simulink model "JenaFox_NCm"  (R2018a)
settings: Solver=ode23s  StartTime=0.0  StopTime=20  MaxStep=maxStep  RelTol=1e-3  AbsTol=absTol
values from neighbouring files (symbols this model uses):
  amplifier = 2.28    [init_motor_parameters.m]
  c_coupling_hip = 7/hip_Ra*hip_k/hip_i    (= 1.22844788155)    [init_motor_parameters.m]
  c_coupling_knee = 7/knee_Ra*knee_k/knee_i    (= 0.698088436179)    [init_motor_parameters.m]
  c_hs = 0.1    [Fox_param.m]
  d_coupling_knee = 0.5    [init_motor_parameters.m]
  d_hs = 0.35    [Fox_param.m]
  g = 9.80665    [Fox_param.m]    (also in init_motor_parameters.m = 9.81)
  hip_i = 1/300.4858    (= 0.00332794428223)    [init_motor_parameters.m]
  hip_Jm = 1/2*hip_m*hip_r^2    (= 1e-07)    [init_motor_parameters.m]
  hip_k = (hip_Um-hip_I0*hip_Ra)*60/(2*pi*hip_n0)    (= 0.00320895298542)    [init_motor_parameters.m]
  hip_Mrg = hip_k*hip_I0g    (= 0.000320895298542)    [init_motor_parameters.m]
  hip_Mrhg = hip_k*hip_Iag    (= 0.000381865405265)    [init_motor_parameters.m]
  hip_na = (hip_Us-(hip_I0*hip_Ra))/hip_k    (= 105.13168591)    [init_motor_parameters.m]
  hip_Ra = hip_Um/hip_Is    (= 5.49450549451)    [init_motor_parameters.m]
  IC_motor_hip_l = deg2rad(IC_phi_hip_l/hip_i)    [init_motor_parameters.m]
  IC_motor_hip_r = deg2rad(IC_phi_hip_r/hip_i)    [init_motor_parameters.m]
  IC_motor_knee_l = deg2rad(IC_phi_knee_l/knee_i)    [init_motor_parameters.m]
  IC_motor_knee_r = deg2rad(IC_phi_knee_r/knee_i)    [init_motor_parameters.m]
  IC_phi_hip_l = 10    [Fox_param.m]
  IC_phi_hip_r = -29    [Fox_param.m]
  IC_v_motor_hip = 0    [init_motor_parameters.m]
  IC_v_motor_knee = 0    [init_motor_parameters.m]
  k_gx = 10*M_RB/0.01    [Fox_param.m]
  k_gy = 150*M_RB/0.01    [Fox_param.m]
  knee_i = 1/185.8428    (= 0.00538089180748)    [init_motor_parameters.m]
  knee_Jm = 1/2*knee_m*knee_r^2    (= 3.2e-08)    [init_motor_parameters.m]
  knee_k = (knee_Um-knee_I0*knee_Ra)*60/(2*pi*knee_n0)    (= 0.000596244182085)    [init_motor_parameters.m]
  knee_Mrg = knee_k*knee_I0g    (= 6.55868600293e-05)    [init_motor_parameters.m]
  knee_Mrhg = knee_k*knee_Iag    (= 9.59953133156e-05)    [init_motor_parameters.m]
  knee_na = (knee_Us-knee_I0*knee_Ra)/knee_k    (= 1360.36733855)    [init_motor_parameters.m]
  knee_Ra = knee_Um/knee_Is    (= 1.11111111111)    [init_motor_parameters.m]
  mu_slide = 4.6    [Fox_param.m]
  mu_stick = 0.8    [Fox_param.m]
  v_gx_max = 0.06    [Fox_param.m]
  v_gy_max = 0.70    (= 0.7)    [Fox_param.m]
  vLimit = 0.01    [Fox_param.m]
undefined symbols (not defined in the file or in its folder): param, smiData, X, Y, Z
libraries: sm_lib x38, nesl_utility x32, simulink x22, simulink_extras x8
(part 1 of 3)
settings Model: SimulationMode=accelerator  Creator=Work  LastModifiedBy=Work
settings RTWCC: Toolchain=MinGW64 | gmake (64-bit Windows)
settings ExplorerConfigSet: SimMechanicsOpenEditorOnUpdate=off  InternalSimMechanicsExplorerSettings="<ExplorerConfiguration><canonicalview>default</canonicalview><AnimationSetting><BasePlaybackSpeed>1.0</BasePlaybackSpeed><PlaybackSpeedFactor>0.0625</PlaybackSpeedFactor></AnimationSetting><TilePanel><TileInfo><Tiles Columns=\"1\" Count=\"1\" Rows=\"1\"><Column Weight=\"1\"/><Row Weight=\"1\"/><Tile Height=\"1\" Width=\"1\" X=\"0\" Y=\"0\"/></Tiles></TileInfo><SceneInfo><SceneViewer><BGColor><R>1</R><G>1</G><B>1</B></BGColor><Camera><DoPerspective>on</DoPerspective><Position><X>-4.33680868994201774e-19</X><Y>0.187999999999999973</Y><Z>0.5</Z></Position><Center><X>-4.33680868994201774e-19</X><Y>0.187999999999999973</Y><Z>-0.5</Z></Center><Up><X>0</X><Y>1</Y><Z>0</Z></Up><ViewLimDist>1</ViewLimDist><YLim>0.466307658154998583</YLim><XLim>0.581939865120500666</XLim></Camera></SceneViewer></SceneInfo></TilePanel><MechEditorPanel><Cameras><Camera><Id>Camera1</Id><Value><Name>Camera1</Name><NativeCamera><PositionTrackingFeature>Subsystem.Camera.Frame1</PositionTrackingFeature><CenterTrackingFeature>Subsystem.Camera.Frame1</CenterTrackingFeature><UpVectorTrackingFeature>Subsystem.Camera.Frame1</UpVectorTrackingFeature><CenterTrackingOrigin>off</CenterTrackingOrigin><CenterTrackingDirection>-Z</CenterTrackingDirection><UpVectorTrackingDirection>+Y</UpVectorTrackingDirection></NativeCamera></Value></Camera></Cameras><GfxPanelCameraMap><MapElement CameraMLId=\"Camera1\" GfxPanelIndex=\"0\"/></GfxPanelCameraMap><VideoCreator><PlaybackSpeedRatio>1.0</PlaybackSpeedRatio><FrameRate>30</FrameRate><VideoFormat>Motion JPEG AVI</VideoFormat><FrameSize>auto</FrameSize></VideoCreator></MechEditorPanel></ExplorerConfiguration>"

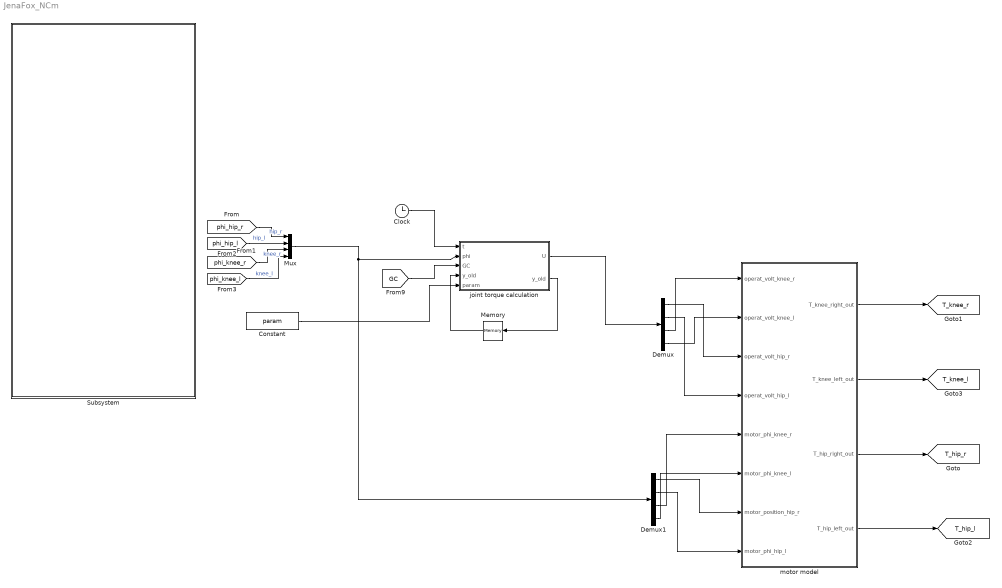
== system JenaFox_NCm ==
  Clock : Clock
  Constant : Constant  Value=param
  Demux : Demux
  Demux1 : Demux
  Memory : Memory  InitialCondition=[0 0;0 0;0 0;0 0;0 0]
  Mux : Mux
  Subsystem : Subsystem
      mask Display: image('robot_new.png');
  joint torque calculation : MATLAB Function  TreatAsAtomicUnit=on  SystemSampleTime=1e-3
  motor model : Subsystem
  tag scope: T_hip_l=global, T_hip_r=global, T_knee_l=global, T_knee_r=global
  wires:
  motor model/2(T_knee_left_out) -> [T_knee_l]
  motor model/1(T_knee_right_out) -> [T_knee_r]
  motor model/4(T_hip_left_out) -> [T_hip_l]
  motor model/3(T_hip_right_out) -> [T_hip_r]
  [phi_knee_l] -> Mux/4  "knee_l"
  [phi_hip_r] -> Mux/1  "hip_r"
  Mux/1 -> joint torque calculation/2(phi), Demux1/1
  [phi_hip_l] -> Mux/2  "hip_l"
  [phi_knee_r] -> Mux/3  "knee_r"
  Demux1/1 -> motor model/7(motor_position_hip_r)
  Demux1/2 -> motor model/8(motor_phi_hip_l)
  Demux1/3 -> motor model/5(motor_phi_knee_r)
  Demux1/4 -> motor model/6(motor_phi_knee_l)
  joint torque calculation/1(U) -> Demux/1
  Demux/1 -> motor model/3(operat_volt_hip_r)
  Demux/2 -> motor model/4(operat_volt_hip_l)
  Demux/3 -> motor model/1(operat_volt_knee_r)
  Demux/4 -> motor model/2(operat_volt_knee_l)
  Clock/1 -> joint torque calculation/1(t)
  [GC] -> joint torque calculation/3(GC)
  joint torque calculation/2(y_old) -> Memory/1
  Memory/1 -> joint torque calculation/4("y_old ")
  Constant/1 -> joint torque calculation/5(param)

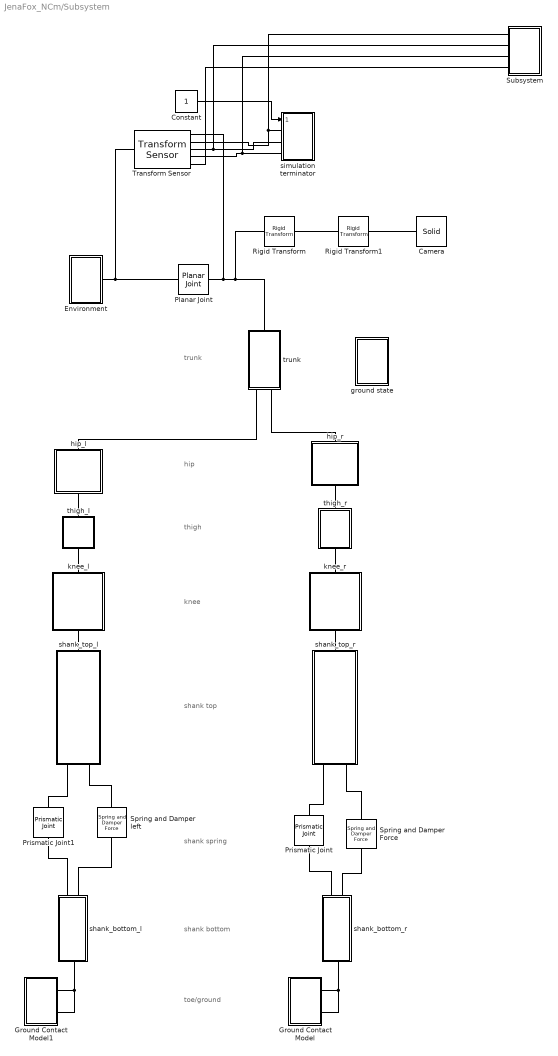
== system JenaFox_NCm/Subsystem ==
  note: trunk
  note: hip
  note: thigh
  note: knee
  note: shank top
  note: shank spring
  note: shank bottom
  note: toe/ground
  Camera : sm_lib/Body Elements/Solid  InertiaType=Custom  Mass=0  MassUnits=kg  CenterOfMass=[0 0 0]  CenterOfMassUnits=m  MomentsOfInertia=[0 0 0]  MomentsOfInertiaUnits=kg*m^2  ProductsOfInertia=[0 0 0]  ProductsOfInertiaUnits=kg*m^2  DensityBased=on  Density=1000  DensityUnits=kg/m^3  DoExposeReferenceFrame=off  SerializedFrames=<Frames><Frame><Id>Frame1</Id><Value><Name>F1</Name><Origin><Source>CenterOfMassFrame</Source><FeatureName></FeatureName></Origin><PrimaryAxis><DefinedDirection>+Z</DefinedDirection><Source>ReferenceFrame</Source><SourceDirection>+Z</SourceDirection><FeatureName></FeatureName></PrimaryAxis><SecondaryAxis><DefinedDirection>+X</DefinedDirection><Source>ReferenceFrame</Source><SourceDirection>+X</SourceDirection><FeatureName></FeatureName></SecondaryAxis></Value></Frame></Frames>  GraphicType=FromGeometry  MarkerShape=Sphere  MarkerSize=10  GraphicVisPropType=SimpleVisualProperties  GraphicDiffuseColor=[0.5 0.5 0.5]  GraphicSpecularColor=[0.5 0.5 0.5 1.0]  GraphicAmbientColor=[0.15 0.15 0.15 1.0]  GraphicEmissiveColor=[0.0 0.0 0.0 1.0]  GraphicShininess=75  GraphicOpacity=1.0  GeometryShape=Sphere  RectangleSize=[1 1]  RectangleSizeUnits=m  BrickDimensions=[1 1 1]  BrickDimensionUnits=m  CylinderRadius=1  CylinderRadiusUnits=m  CylinderLength=1  CylinderLengthUnits=m  SphereRadius=1e-6  SphereRadiusUnits=m  EllipsoidRadii=[1 1 1]  EllipsoidRadiiUnits=m  ExtrusionCrossSection=[1 1; -1 1; -1 -1; 1 -1]  ExtrusionCrossSectionUnits=m  ExtrusionLength=1  ExtrusionLengthUnits=m  PolygonNumSides=3  PolygonOuterRadius=1  PolygonOuterRadiusUnits=m  ExtGeomFileType=STEP  ExtGeomFileUnits=m  RevolutionCrossSection=[1 1; 1 -1; 2 -1; 2 1]  RevolutionCrossSectionUnits=m  RevolutionExtent=Full  RevolutionAngle=180  RevolutionAngleUnits=deg
  Constant : Constant
  Environment : Subsystem
  Ground Contact Model : Subsystem
  Ground Contact Model1 : Subsystem
  Planar Joint : sm_lib/Joints/Planar Joint  SenseConstraintForce=off  SenseConstraintForceX=off  SenseConstraintForceY=off  SenseConstraintForceZ=off  SenseConstraintTorque=off  SenseConstraintTorqueX=off  SenseConstraintTorqueY=off  SenseConstraintTorqueZ=off  SenseTotalForce=off  SenseTotalForceX=off  SenseTotalForceY=off  SenseTotalForceZ=off  SenseTotalTorque=off  SenseTotalTorqueX=off  SenseTotalTorqueY=off  SenseTotalTorqueZ=off  CompositeWrenchDir=FollowerOnBase  CompositeWrenchFrame=BaseFrame  PxEquilibriumPosition=0  PxEquilibriumPositionUnits=m  PxSpringStiffness=0  PxSpringStiffnessUnits=N/m  PxDampingCoefficient=0  PxDampingCoefficientUnits=N/(m/s)  PxTorqueActuationMode=NoTorque  PxMotionActuationMode=ComputedMotion  PxSensePosition=off  PxSenseVelocity=off  PxSenseAcceleration=off  PxSenseTorqueForce=off  PxPositionTargetSpecify=off  PxPositionTargetPriority=High  PxPositionTargetValue=0  PxPositionTargetValueUnits=m  PxVelocityTargetSpecify=on  PxVelocityTargetPriority=High  PxVelocityTargetValue=IC_vCOM_x  PxVelocityTargetValueUnits=m/s  PyEquilibriumPosition=0  PyEquilibriumPositionUnits=m  PySpringStiffness=0  PySpringStiffnessUnits=N/m  PyDampingCoefficient=0  PyDampingCoefficientUnits=N/(m/s)  PyTorqueActuationMode=NoTorque  PyMotionActuationMode=ComputedMotion  PySensePosition=off  PySenseVelocity=off  PySenseAcceleration=off  PySenseTorqueForce=off  PyPositionTargetSpecify=on  PyPositionTargetPriority=High  PyPositionTargetValue=IC_y  PyPositionTargetValueUnits=m  PyVelocityTargetSpecify=on  PyVelocityTargetPriority=High  PyVelocityTargetValue=IC_vCOM_y  PyVelocityTargetValueUnits=m/s  RzEquilibriumPosition=0  RzEquilibriumPositionUnits=deg  RzSpringStiffness=500  RzSpringStiffnessUnits=N*m/deg  RzDampingCoefficient=5  RzDampingCoefficientUnits=N*m/(deg/s)  RzTorqueActuationMode=NoTorque  RzMotionActuationMode=ComputedMotion  RzSensePosition=off  RzSenseVelocity=off  RzSenseAcceleration=off  RzSenseTorqueForce=off  RzPositionTargetSpecify=on  RzPositionTargetPriority=High  RzPositionTargetValue=0  RzPositionTargetValueUnits=deg  RzVelocityTargetSpecify=on  RzVelocityTargetPriority=High  RzVelocityTargetValue=0  RzVelocityTargetValueUnits=deg/s
  Prismatic Joint : sm_lib/Joints/Prismatic Joint  SenseConstraintForce=off  SenseConstraintForceX=off  SenseConstraintForceY=off  SenseConstraintForceZ=off  SenseConstraintTorque=off  SenseConstraintTorqueX=off  SenseConstraintTorqueY=off  SenseConstraintTorqueZ=off  SenseTotalForce=off  SenseTotalForceX=off  SenseTotalForceY=off  SenseTotalForceZ=off  SenseTotalTorque=off  SenseTotalTorqueX=off  SenseTotalTorqueY=off  SenseTotalTorqueZ=off  CompositeWrenchDir=FollowerOnBase  CompositeWrenchFrame=BaseFrame  EquilibriumPosition=0  EquilibriumPositionUnits=m  SpringStiffness=0  SpringStiffnessUnits=N/m  DampingCoefficient=0  DampingCoefficientUnits=N/(m/s)  TorqueActuationMode=NoTorque  MotionActuationMode=ComputedMotion  SensePosition=off  SenseVelocity=off  SenseAcceleration=off  SenseTorqueForce=off  PositionTargetSpecify=off  PositionTargetPriority=High  PositionTargetValue=0  PositionTargetValueUnits=m  VelocityTargetSpecify=off  VelocityTargetPriority=High  VelocityTargetValue=0  VelocityTargetValueUnits=m/s
  Prismatic Joint1 : sm_lib/Joints/Prismatic Joint  SenseConstraintForce=off  SenseConstraintForceX=off  SenseConstraintForceY=off  SenseConstraintForceZ=off  SenseConstraintTorque=off  SenseConstraintTorqueX=off  SenseConstraintTorqueY=off  SenseConstraintTorqueZ=off  SenseTotalForce=off  SenseTotalForceX=off  SenseTotalForceY=off  SenseTotalForceZ=off  SenseTotalTorque=off  SenseTotalTorqueX=off  SenseTotalTorqueY=off  SenseTotalTorqueZ=off  CompositeWrenchDir=FollowerOnBase  CompositeWrenchFrame=BaseFrame  EquilibriumPosition=0  EquilibriumPositionUnits=m  SpringStiffness=0  SpringStiffnessUnits=N/m  DampingCoefficient=0  DampingCoefficientUnits=N/(m/s)  TorqueActuationMode=NoTorque  MotionActuationMode=ComputedMotion  SensePosition=off  SenseVelocity=off  SenseAcceleration=off  SenseTorqueForce=off  PositionTargetSpecify=off  PositionTargetPriority=High  PositionTargetValue=0  PositionTargetValueUnits=m  VelocityTargetSpecify=off  VelocityTargetPriority=High  VelocityTargetValue=0  VelocityTargetValueUnits=m/s
  Rigid Transform : sm_lib/Frames and Transforms/Rigid Transform  TranslationMethod=StandardAxis  TranslationStandardOffset=.5  TranslationLengthUnit=m  TranslationStandardAxis=+Z  TranslationCartesianOffset=[0 0 0]  TranslationROffset=0  TranslationROffsetUnits=m  TranslationZOffset=0  TranslationZOffsetUnits=m  TranslationThetaOffset=0  TranslationThetaOffsetUnits=deg  RotationMethod=None  RotationAngleUnits=deg  RotationStandardAxis=+Z  RotationAngle=0.0  RotationArbitraryAxis=[0 0 1]  FollAlignAxisA=+X  BaseAlignAxisA=+Y  FollAlignAxisB=+Y  BaseAlignAxisB=+Z  RotationSequenceAxes=FollowerAxes  RotationSequence=XYX  RotationSequenceAngles=[0 0 0]  RotationSequenceAnglesUnits=deg  RotationMatrix=[1 0 0; 0 1 0; 0 0 1]
  Rigid Transform1 : sm_lib/Frames and Transforms/Rigid Transform  TranslationMethod=StandardAxis  TranslationStandardOffset=.1  TranslationLengthUnit=m  TranslationStandardAxis=-Y  TranslationCartesianOffset=[0 0 0]  TranslationROffset=0  TranslationROffsetUnits=m  TranslationZOffset=0  TranslationZOffsetUnits=m  TranslationThetaOffset=0  TranslationThetaOffsetUnits=deg  RotationMethod=None  RotationAngleUnits=deg  RotationStandardAxis=+Z  RotationAngle=0.0  RotationArbitraryAxis=[0 0 1]  FollAlignAxisA=+X  BaseAlignAxisA=+Y  FollAlignAxisB=+Y  BaseAlignAxisB=+Z  RotationSequenceAxes=FollowerAxes  RotationSequence=XYX  RotationSequenceAngles=[0 0 0]  RotationSequenceAnglesUnits=deg  RotationMatrix=[1 0 0; 0 1 0; 0 0 1]
  Spring and Damper Force : sm_lib/Forces and Torques/Spring and Damper Force  NaturalLength=spring_ankle_rl_r  NaturalLengthUnits=m  SpringStiffness=spring_ankle_c_r  SpringStiffnessUnits=N/m  DampingCoefficient=damper_ankle_r  DampingCoefficientUnits=N/(m/s)  SenseForce=off
      settings: SourceProductName=Simscape Multibody
  Spring and Damper left : sm_lib/Forces and Torques/Spring and Damper Force  NaturalLength=spring_ankle_rl_l  NaturalLengthUnits=m  SpringStiffness=spring_ankle_c_l  SpringStiffnessUnits=N/m  DampingCoefficient=damper_ankle_l  DampingCoefficientUnits=N/(m/s)  SenseForce=off
      settings: SourceProductName=Simscape Multibody
  Subsystem : Subsystem
  Transform Sensor : sm_lib/Frames and Transforms/Transform Sensor  MeasurementFrame=World  SenseAngle=off  SenseAxis=off  SenseAngle1=off  SenseAngle2=off  SenseAngle3=off  SenseQ=off  SenseR=off  SenseOmegaX=off  SenseOmegaY=off  SenseOmegaZ=off  SenseOmega1=off  SenseOmega2=off  SenseOmega3=off  SenseQDot=off  SenseRDot=off  SenseAlphaX=off  SenseAlphaY=off  SenseAlphaZ=off  SenseAlpha1=off  SenseAlpha2=off  SenseAlpha3=off  SenseQDDot=off  SenseRDDot=off  SenseX=on  SenseY=on  SenseZ=off  SenseRad=off  SenseAzim=off  SenseDist=off  SenseInc=off  SenseXDot=on  SenseYDot=on  SenseZDot=off  SenseRadDot=off  SenseAzimDot=off  SenseDistDot=off  SenseIncDot=off  SenseXDDot=off  SenseYDDot=off  SenseZDDot=off  SenseRadDDot=off  SenseAzimDDot=off  SenseDistDDot=off  SenseIncDDot=off
  ground state : Subsystem
  hip_l : Subsystem
  hip_r : Subsystem
  knee_l : Subsystem
  knee_r : Subsystem
  shank_bottom_l : Subsystem
  shank_bottom_r : Subsystem
  shank_top_l : Subsystem
  shank_top_r : Subsystem
  simulation terminator : Subsystem
  thigh_l : Subsystem
  thigh_r : Subsystem
  trunk : Subsystem
  wires:
  Constant/1 -> simulation terminator/1(enable)
  connections:
  Spring and Damper Force/LConn1 -- shank_bottom_r/LConn2
  knee_r/RConn1 -- shank_top_r/LConn1
  hip_r/RConn1 -- thigh_r/LConn1
  knee_r/LConn1 -- thigh_r/RConn1
  Prismatic Joint1/LConn1 -- shank_bottom_l/LConn1
  hip_l/RConn1 -- thigh_l/LConn1
  Ground Contact Model/RConn1 -- Ground Contact Model/RConn2 -- shank_bottom_r/RConn1
  Prismatic Joint/RConn1 -- shank_top_r/RConn1
  knee_l/LConn1 -- thigh_l/RConn1
  Spring and Damper left/LConn1 -- shank_bottom_l/LConn2
  Prismatic Joint1/RConn1 -- shank_top_l/RConn1
  Prismatic Joint/LConn1 -- shank_bottom_r/LConn1
  Ground Contact Model1/RConn2 -- Ground Contact Model1/RConn1 -- shank_bottom_l/RConn1
  Spring and Damper left/RConn1 -- shank_top_l/RConn2
  hip_r/LConn1 -- trunk/RConn2
  trunk/RConn1 -- hip_l/LConn1
  Spring and Damper Force/RConn1 -- shank_top_r/RConn2
  shank_top_l/LConn1 -- knee_l/RConn1
  Planar Joint/RConn1 -- Transform Sensor/RConn1 -- Rigid Transform/LConn1 -- trunk/LConn1
  Environment/RConn1 -- Planar Joint/LConn1 -- Transform Sensor/LConn1
  Camera/LConn1 -- Rigid Transform1/RConn1
  Rigid Transform1/LConn1 -- Rigid Transform/RConn1
  simulation terminator/LConn1 -- Subsystem/LConn1 -- Transform Sensor/RConn2
  simulation terminator/LConn2 -- Subsystem/LConn2 -- Transform Sensor/RConn3
  simulation terminator/LConn3 -- Subsystem/LConn3 -- Transform Sensor/RConn4
  Subsystem/LConn4 -- Transform Sensor/RConn5

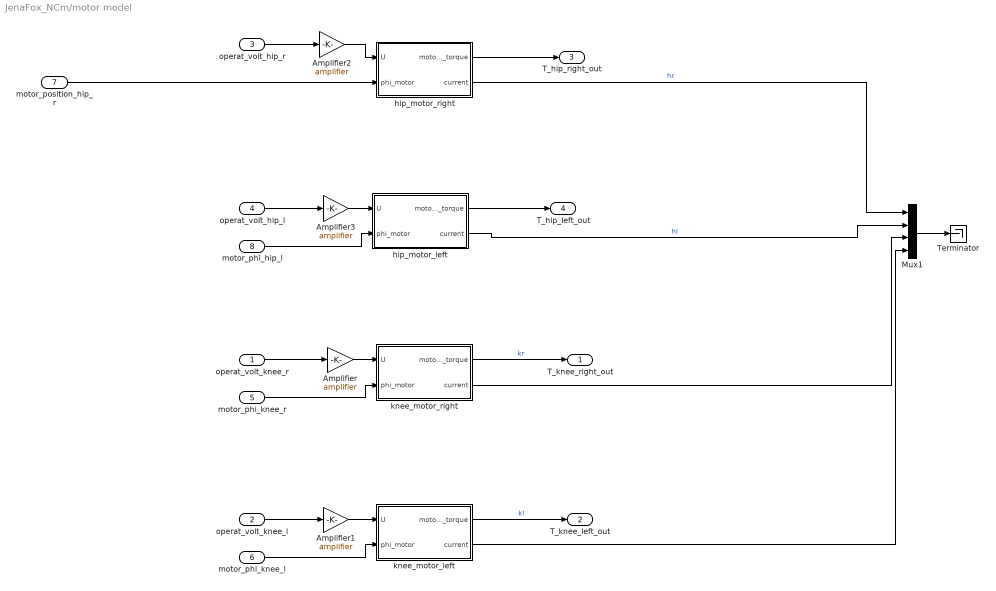
== system JenaFox_NCm/motor model ==
  operat_volt_knee_r : Inport
  operat_volt_knee_l : Inport  Port=2
  operat_volt_hip_r : Inport  Port=3
  operat_volt_hip_l : Inport  Port=4
  motor_phi_knee_r : Inport  Port=5
  motor_phi_knee_l : Inport  Port=6
  motor_position_hip_r : Inport  Port=7
  motor_phi_hip_l : Inport  Port=8
  Amplifier{,1..3} (4 alike) : Gain  Gain=amplifier
  Mux1 : Mux
  Terminator : Terminator
  hip_motor_left : Subsystem  mask(Hip Motor){IC_phi_motor_hip=IC_motor_hip_l}
      mask prompts: IC_phi_motor_hip "Initial position"
  hip_motor_right : Subsystem  mask(Hip Motor){IC_phi_motor_hip=IC_motor_hip_r}
      mask prompts: IC_phi_motor_hip "Initial position"
  knee_motor_left : Subsystem  mask{IC_phi_motor_knee=IC_motor_knee_l}
      mask prompts: IC_phi_motor_knee "Initial motor position"
  knee_motor_right : Subsystem  mask{IC_phi_motor_knee=IC_motor_knee_r}
      mask prompts: IC_phi_motor_knee "Initial motor position"
  T_knee_right_out : Outport
  T_knee_left_out : Outport  Port=2
  T_hip_right_out : Outport  Port=3
  T_hip_left_out : Outport  Port=4
  wires:
  hip_motor_right/1(motor_torque) -> T_hip_right_out/1
  motor_position_hip_r/1 -> hip_motor_right/2(phi_motor)
  Amplifier3/1 -> hip_motor_left/1(U)
  Amplifier2/1 -> hip_motor_right/1(U)
  Amplifier1/1 -> knee_motor_left/1(U)
  Amplifier/1 -> knee_motor_right/1(U)
  operat_volt_hip_l/1 -> Amplifier3/1
  motor_phi_knee_r/1 -> knee_motor_right/2(phi_motor)
  operat_volt_knee_r/1 -> Amplifier/1
  motor_phi_knee_l/1 -> knee_motor_left/2(phi_motor)
  operat_volt_knee_l/1 -> Amplifier1/1
  operat_volt_hip_r/1 -> Amplifier2/1
  motor_phi_hip_l/1 -> hip_motor_left/2(phi_motor)
  knee_motor_right/1(motor_torque) -> T_knee_right_out/1  "kr"
  hip_motor_left/1(motor_torque) -> T_hip_left_out/1
  knee_motor_left/1(motor_torque) -> T_knee_left_out/1  "kl"
  hip_motor_right/2(current) -> Mux1/1  "hr"
  hip_motor_left/2(current) -> Mux1/2  "hl"
  Mux1/1 -> Terminator/1
  knee_motor_right/2(current) -> Mux1/3
  knee_motor_left/2(current) -> Mux1/4

== system JenaFox_NCm/Subsystem/Environment ==
  Ground : sm_lib/Body Elements/Solid  InertiaType=Custom  Mass=0  MassUnits=kg  CenterOfMass=[0 0 0]  CenterOfMassUnits=m  MomentsOfInertia=[0 0 0]  MomentsOfInertiaUnits=kg*m^2  ProductsOfInertia=[0 0 0]  ProductsOfInertiaUnits=kg*m^2  DensityBased=on  Density=1000  DensityUnits=kg/m^3  DoExposeReferenceFrame=on  SerializedFrames=<Frames/>  GraphicType=FromGeometry  MarkerShape=Sphere  MarkerSize=10  GraphicVisPropType=SimpleVisualProperties  GraphicDiffuseColor=[0.5 0.5 0.5]  GraphicSpecularColor=[0.5 0.5 0.5 1.0]  GraphicAmbientColor=[0.15 0.15 0.15 1.0]  GraphicEmissiveColor=[0.0 0.0 0.0 1.0]  GraphicShininess=75  GraphicOpacity=1.0  GeometryShape=Brick  RectangleSize=[1 1]  RectangleSizeUnits=m  BrickDimensions=[100 1e-3 .2]  BrickDimensionUnits=m  CylinderRadius=1  CylinderRadiusUnits=m  CylinderLength=1  CylinderLengthUnits=m  SphereRadius=1  SphereRadiusUnits=m  EllipsoidRadii=[1 1 1]  EllipsoidRadiiUnits=m  ExtrusionCrossSection=[1 1; -1 1; -1 -1; 1 -1]  ExtrusionCrossSectionUnits=m  ExtrusionLength=1  ExtrusionLengthUnits=m  PolygonNumSides=3  PolygonOuterRadius=1  PolygonOuterRadiusUnits=m  ExtGeomFileType=STEP  ExtGeomFileUnits=m  RevolutionCrossSection=[1 1; 1 -1; 2 -1; 2 1]  RevolutionCrossSectionUnits=m  RevolutionExtent=Full  RevolutionAngle=180  RevolutionAngleUnits=deg
  Ground1 : sm_lib/Body Elements/Solid  InertiaType=Custom  Mass=0  MassUnits=kg  CenterOfMass=[0 0 0]  CenterOfMassUnits=m  MomentsOfInertia=[0 0 0]  MomentsOfInertiaUnits=kg*m^2  ProductsOfInertia=[0 0 0]  ProductsOfInertiaUnits=kg*m^2  DensityBased=on  Density=1000  DensityUnits=kg/m^3  DoExposeReferenceFrame=off  SerializedFrames=<Frames><Frame><Id>Frame1</Id><Value><Name>F1</Name><Origin><Source>GeometricFeature</Source><FeatureName>+x -y +z point</FeatureName></Origin><PrimaryAxis><DefinedDirection>+Z</DefinedDirection><Source>ReferenceFrame</Source><SourceDirection>+Z</SourceDirection><FeatureName></FeatureName></PrimaryAxis><SecondaryAxis><DefinedDirection>+X</DefinedDirection><Source>ReferenceFrame</Source><SourceDirection>+X</SourceDirection><FeatureName></FeatureName></SecondaryAxis></Value></Frame></Frames>  GraphicType=FromGeometry  MarkerShape=Cube  MarkerSize=100  GraphicVisPropType=AdvancedVisualProperties  GraphicDiffuseColor=[1 0 0]  GraphicSpecularColor=[0.5 0.5 0.5 1.0]  GraphicAmbientColor=[0.15 0.15 0.15 1.0]  GraphicEmissiveColor=[0.0 0.0 0.0 1.0]  GraphicShininess=75  GraphicOpacity=1.0  GeometryShape=Brick  RectangleSize=[1 1]  RectangleSizeUnits=m  BrickDimensions=[0.1 0.5 0.1]  BrickDimensionUnits=m  CylinderRadius=1  CylinderRadiusUnits=m  CylinderLength=1  CylinderLengthUnits=m  SphereRadius=1  SphereRadiusUnits=m  EllipsoidRadii=[1 1 1]  EllipsoidRadiiUnits=m  ExtrusionCrossSection=[1 1; -1 1; -1 -1; 1 -1]  ExtrusionCrossSectionUnits=m  ExtrusionLength=1  ExtrusionLengthUnits=m  PolygonNumSides=3  PolygonOuterRadius=1  PolygonOuterRadiusUnits=m  ExtGeomFileType=STEP  ExtGeomFileUnits=m  RevolutionCrossSection=[1 1; 1 -1; 2 -1; 2 1]  RevolutionCrossSectionUnits=m  RevolutionExtent=Full  RevolutionAngle=180  RevolutionAngleUnits=deg
  Ground2 : sm_lib/Body Elements/Solid  InertiaType=Custom  Mass=0  MassUnits=kg  CenterOfMass=[0 0 0]  CenterOfMassUnits=m  MomentsOfInertia=[0 0 0]  MomentsOfInertiaUnits=kg*m^2  ProductsOfInertia=[0 0 0]  ProductsOfInertiaUnits=kg*m^2  DensityBased=on  Density=1000  DensityUnits=kg/m^3  DoExposeReferenceFrame=off  SerializedFrames=<Frames><Frame><Id>Frame1</Id><Value><Name>F1</Name><Origin><Source>GeometricFeature</Source><FeatureName>+x -y +z point</FeatureName></Origin><PrimaryAxis><DefinedDirection>+Z</DefinedDirection><Source>ReferenceFrame</Source><SourceDirection>+Z</SourceDirection><FeatureName></FeatureName></PrimaryAxis><SecondaryAxis><DefinedDirection>+X</DefinedDirection><Source>ReferenceFrame</Source><SourceDirection>+X</SourceDirection><FeatureName></FeatureName></SecondaryAxis></Value></Frame></Frames>  GraphicType=FromGeometry  MarkerShape=Cube  MarkerSize=100  GraphicVisPropType=AdvancedVisualProperties  GraphicDiffuseColor=[1 0 0]  GraphicSpecularColor=[0.5 0.5 0.5 1.0]  GraphicAmbientColor=[0.15 0.15 0.15 1.0]  GraphicEmissiveColor=[0.0 0.0 0.0 1.0]  GraphicShininess=75  GraphicOpacity=1.0  GeometryShape=Brick  RectangleSize=[1 1]  RectangleSizeUnits=m  BrickDimensions=[0.1 0.5 0.1]  BrickDimensionUnits=m  CylinderRadius=1  CylinderRadiusUnits=m  CylinderLength=1  CylinderLengthUnits=m  SphereRadius=1  SphereRadiusUnits=m  EllipsoidRadii=[1 1 1]  EllipsoidRadiiUnits=m  ExtrusionCrossSection=[1 1; -1 1; -1 -1; 1 -1]  ExtrusionCrossSectionUnits=m  ExtrusionLength=1  ExtrusionLengthUnits=m  PolygonNumSides=3  PolygonOuterRadius=1  PolygonOuterRadiusUnits=m  ExtGeomFileType=STEP  ExtGeomFileUnits=m  RevolutionCrossSection=[1 1; 1 -1; 2 -1; 2 1]  RevolutionCrossSectionUnits=m  RevolutionExtent=Full  RevolutionAngle=180  RevolutionAngleUnits=deg
  Mechanism Configuration : sm_lib/Utilities/Mechanism Configuration  UniformGravity=Constant  GravityVector=[0 -g 0]  GravityUnits=m/s^2  LinearizationDelta=0.001
  Rigid Transform : sm_lib/Frames and Transforms/Rigid Transform  TranslationMethod=Cartesian  TranslationStandardOffset=0  TranslationLengthUnit=m  TranslationStandardAxis=+Z  TranslationCartesianOffset=[0 0 0]  TranslationROffset=0  TranslationROffsetUnits=m  TranslationZOffset=0  TranslationZOffsetUnits=m  TranslationThetaOffset=0  TranslationThetaOffsetUnits=deg  RotationMethod=None  RotationAngleUnits=deg  RotationStandardAxis=+Z  RotationAngle=0.0  RotationArbitraryAxis=[0 0 1]  FollAlignAxisA=+X  BaseAlignAxisA=+Y  FollAlignAxisB=+Y  BaseAlignAxisB=+Z  RotationSequenceAxes=FollowerAxes  RotationSequence=XYX  RotationSequenceAngles=[0 0 0]  RotationSequenceAnglesUnits=deg  RotationMatrix=[1 0 0; 0 1 0; 0 0 1]
  Rigid Transform1 : sm_lib/Frames and Transforms/Rigid Transform  TranslationMethod=Cartesian  TranslationStandardOffset=0  TranslationLengthUnit=m  TranslationStandardAxis=+Z  TranslationCartesianOffset=[5 0 -0.1]  TranslationROffset=0  TranslationROffsetUnits=m  TranslationZOffset=0  TranslationZOffsetUnits=m  TranslationThetaOffset=0  TranslationThetaOffsetUnits=deg  RotationMethod=None  RotationAngleUnits=deg  RotationStandardAxis=+Z  RotationAngle=0.0  RotationArbitraryAxis=[0 0 1]  FollAlignAxisA=+X  BaseAlignAxisA=+Y  FollAlignAxisB=+Y  BaseAlignAxisB=+Z  RotationSequenceAxes=FollowerAxes  RotationSequence=XYX  RotationSequenceAngles=[0 0 0]  RotationSequenceAnglesUnits=deg  RotationMatrix=[1 0 0; 0 1 0; 0 0 1]
  Rigid Transform2 : sm_lib/Frames and Transforms/Rigid Transform  TranslationMethod=Cartesian  TranslationStandardOffset=0  TranslationLengthUnit=m  TranslationStandardAxis=+Z  TranslationCartesianOffset=[5 0 0]  TranslationROffset=0  TranslationROffsetUnits=m  TranslationZOffset=0  TranslationZOffsetUnits=m  TranslationThetaOffset=0  TranslationThetaOffsetUnits=deg  RotationMethod=None  RotationAngleUnits=deg  RotationStandardAxis=+Z  RotationAngle=0.0  RotationArbitraryAxis=[0 0 1]  FollAlignAxisA=+X  BaseAlignAxisA=+Y  FollAlignAxisB=+Y  BaseAlignAxisB=+Z  RotationSequenceAxes=FollowerAxes  RotationSequence=XYX  RotationSequenceAngles=[0 0 0]  RotationSequenceAnglesUnits=deg  RotationMatrix=[1 0 0; 0 1 0; 0 0 1]
  Solver Configuration1 : nesl_utility/Solver Configuration  PhysicalDomain=network_engine_domain  SubClassName=solver  LeftPortType=input  RightPortType=generic  Tones=[]  Harmonics=[]  SimulateNoise=off  Profile=off  UseLocalSampling=off  EnableSwitchedLinearOptims=on  FrequencyDomain=off  UseCCode=off  RelTol=0.001  AbsTol=1e-06  MinStep=1e-09  ToWorkspace=off  RevertToSquareIcSolve=off  NumHomotopyIterations=100  PhasorMode=off  PhasorModeNumHarmonics=1  DoDC=off  ResidualTolerance=1e-09  UseLocalSolver=off  LocalSolverChoice=NE_BACKWARD_EULER_ADVANCER  LocalSolverSampleTime=0.001  DoFixedCost=off  MaxNonlinIter=3  MaxModeIter=2  LinearAlgebra=Sparse  EquationFormulation=NE_TIME_EF  DelaysMemoryBudget=1024  AutomaticFiltering=on  FilteringTimeConstant=0.001
  World Frame X-forward Y-lateral Z-up : sm_lib/Frames and Transforms/World Frame
  Conn1 : PMIOPort  Side=Right
  connections:
  Solver Configuration1/RConn1 -- Rigid Transform1/LConn1 -- Ground/RConn1 -- World Frame X-forward Y-lateral Z-up/RConn1 -- Rigid Transform/LConn1 -- Mechanism Configuration/RConn1
  Rigid Transform/RConn1 -- Conn1/RConn1
  Rigid Transform1/RConn1 -- Ground1/LConn1 -- Rigid Transform2/LConn1
  Ground2/LConn1 -- Rigid Transform2/RConn1

== system JenaFox_NCm/Subsystem/Ground Contact Model ==
  External Force and Torque : sm_lib/Forces and Torques/External Force and Torque  ForceResolutionFrame=World  EnableForceX=on  EnableForceY=on  EnableForceZ=off  EnableForce=off  TorqueResolutionFrame=AttachedFrame  EnableTorqueX=off  EnableTorqueY=off  EnableTorqueZ=off  EnableTorque=off
  Ground Friction Model : Subsystem
  PS-Simulink Converter : nesl_utility/PS-Simulink Converter  PhysicalDomain=network_engine_domain  SubClassName=ps_output  LeftPortType=input  RightPortType=output  PseudoPeriodic=off  Frequencies=[]  Unit=m  AffineConversion=off
  PS-Simulink Converter1 : nesl_utility/PS-Simulink Converter  PhysicalDomain=network_engine_domain  SubClassName=ps_output  LeftPortType=input  RightPortType=output  PseudoPeriodic=off  Frequencies=[]  Unit=m/s  AffineConversion=off
  PS-Simulink Converter2 : nesl_utility/PS-Simulink Converter  PhysicalDomain=network_engine_domain  SubClassName=ps_output  LeftPortType=input  RightPortType=output  PseudoPeriodic=off  Frequencies=[]  Unit=m  AffineConversion=off
  PS-Simulink Converter3 : nesl_utility/PS-Simulink Converter  PhysicalDomain=network_engine_domain  SubClassName=ps_output  LeftPortType=input  RightPortType=output  PseudoPeriodic=off  Frequencies=[]  Unit=m/s  AffineConversion=off
  Scope : Scope
  Simulink-PS Converter : nesl_utility/Simulink-PS Converter  PhysicalDomain=network_engine_domain  SubClassName=ps_input  LeftPortType=input  RightPortType=output  PseudoPeriodic=off  Frequencies=[]  NoiseDistribution=none  NoiseParameters=[]  Unit=1  AffineConversion=off  FilteringAndDerivatives=zero  SimscapeFilterOrder=1  InputFilterTimeConstant=0.001  UdotUserProvided=1
  Simulink-PS Converter1 : nesl_utility/Simulink-PS Converter  PhysicalDomain=network_engine_domain  SubClassName=ps_input  LeftPortType=input  RightPortType=output  PseudoPeriodic=off  Frequencies=[]  NoiseDistribution=none  NoiseParameters=[]  Unit=1  AffineConversion=off  FilteringAndDerivatives=zero  SimscapeFilterOrder=1  InputFilterTimeConstant=0.001  UdotUserProvided=1
  Terminator : Terminator
  Transform Sensor : sm_lib/Frames and Transforms/Transform Sensor  MeasurementFrame=World  SenseAngle=off  SenseAxis=off  SenseAngle1=off  SenseAngle2=off  SenseAngle3=off  SenseQ=off  SenseR=off  SenseOmegaX=off  SenseOmegaY=off  SenseOmegaZ=off  SenseOmega1=off  SenseOmega2=off  SenseOmega3=off  SenseQDot=off  SenseRDot=off  SenseAlphaX=off  SenseAlphaY=off  SenseAlphaZ=off  SenseAlpha1=off  SenseAlpha2=off  SenseAlpha3=off  SenseQDDot=off  SenseRDDot=off  SenseX=on  SenseY=on  SenseZ=off  SenseRad=off  SenseAzim=off  SenseDist=off  SenseInc=off  SenseXDot=on  SenseYDot=on  SenseZDot=off  SenseRadDot=off  SenseAzimDot=off  SenseDistDot=off  SenseIncDot=off  SenseXDDot=off  SenseYDDot=off  SenseZDDot=off  SenseRadDDot=off  SenseAzimDDot=off  SenseDistDDot=off  SenseIncDDot=off
  World Frame : sm_lib/Frames and Transforms/World Frame
  contact? : simulink/Logic and Bit Operations/Compare To Zero  relop=<=  OutDataTypeStr=boolean
  Toe : PMIOPort  Side=Right
  GRF : PMIOPort  Port=2  Side=Right
  tag scope: GC_r=global
  wires:
  PS-Simulink Converter/1 -> contact?/1, Ground Friction Model/1(dy [m])  "yBall left"
  contact?/1 -> Ground Friction Model/Enable, [GC_r]
  Ground Friction Model/3(Stiction!) -> Terminator/1
  PS-Simulink Converter3/1 -> Ground Friction Model/4(vx [m/s])
  PS-Simulink Converter2/1 -> Ground Friction Model/3(x [m])
  PS-Simulink Converter1/1 -> Ground Friction Model/2(vy [m/s])
  Ground Friction Model/2(Fx_Friction [N]) -> Simulink-PS Converter/1
  Ground Friction Model/1(Fy_Ground[N]) -> Scope/1, Simulink-PS Converter1/1
  connections:
  Transform Sensor/RConn2 -- PS-Simulink Converter2/LConn1
  External Force and Torque/RConn1 -- GRF/RConn1
  Transform Sensor/RConn1 -- Toe/RConn1
  Transform Sensor/RConn3 -- PS-Simulink Converter/LConn1
  Transform Sensor/RConn5 -- PS-Simulink Converter1/LConn1
  Transform Sensor/LConn1 -- World Frame/RConn1
  Transform Sensor/RConn4 -- PS-Simulink Converter3/LConn1
  External Force and Torque/LConn2 -- Simulink-PS Converter1/RConn1
  External Force and Torque/LConn1 -- Simulink-PS Converter/RConn1

== system JenaFox_NCm/Subsystem/Ground Contact Model1 ==
  External Force and Torque : sm_lib/Forces and Torques/External Force and Torque  ForceResolutionFrame=World  EnableForceX=on  EnableForceY=on  EnableForceZ=off  EnableForce=off  TorqueResolutionFrame=AttachedFrame  EnableTorqueX=off  EnableTorqueY=off  EnableTorqueZ=off  EnableTorque=off
  Ground Friction Model : Subsystem
  PS-Simulink Converter : nesl_utility/PS-Simulink Converter  PhysicalDomain=network_engine_domain  SubClassName=ps_output  LeftPortType=input  RightPortType=output  PseudoPeriodic=off  Frequencies=[]  Unit=m  AffineConversion=off
  PS-Simulink Converter1 : nesl_utility/PS-Simulink Converter  PhysicalDomain=network_engine_domain  SubClassName=ps_output  LeftPortType=input  RightPortType=output  PseudoPeriodic=off  Frequencies=[]  Unit=m/s  AffineConversion=off
  PS-Simulink Converter2 : nesl_utility/PS-Simulink Converter  PhysicalDomain=network_engine_domain  SubClassName=ps_output  LeftPortType=input  RightPortType=output  PseudoPeriodic=off  Frequencies=[]  Unit=m  AffineConversion=off
  PS-Simulink Converter3 : nesl_utility/PS-Simulink Converter  PhysicalDomain=network_engine_domain  SubClassName=ps_output  LeftPortType=input  RightPortType=output  PseudoPeriodic=off  Frequencies=[]  Unit=m/s  AffineConversion=off
  Scope : Scope
  Simulink-PS Converter : nesl_utility/Simulink-PS Converter  PhysicalDomain=network_engine_domain  SubClassName=ps_input  LeftPortType=input  RightPortType=output  PseudoPeriodic=off  Frequencies=[]  NoiseDistribution=none  NoiseParameters=[]  Unit=1  AffineConversion=off  FilteringAndDerivatives=zero  SimscapeFilterOrder=1  InputFilterTimeConstant=0.001  UdotUserProvided=1
  Simulink-PS Converter1 : nesl_utility/Simulink-PS Converter  PhysicalDomain=network_engine_domain  SubClassName=ps_input  LeftPortType=input  RightPortType=output  PseudoPeriodic=off  Frequencies=[]  NoiseDistribution=none  NoiseParameters=[]  Unit=1  AffineConversion=off  FilteringAndDerivatives=zero  SimscapeFilterOrder=1  InputFilterTimeConstant=0.001  UdotUserProvided=1
  Terminator : Terminator
  Transform Sensor : sm_lib/Frames and Transforms/Transform Sensor  MeasurementFrame=World  SenseAngle=off  SenseAxis=off  SenseAngle1=off  SenseAngle2=off  SenseAngle3=off  SenseQ=off  SenseR=off  SenseOmegaX=off  SenseOmegaY=off  SenseOmegaZ=off  SenseOmega1=off  SenseOmega2=off  SenseOmega3=off  SenseQDot=off  SenseRDot=off  SenseAlphaX=off  SenseAlphaY=off  SenseAlphaZ=off  SenseAlpha1=off  SenseAlpha2=off  SenseAlpha3=off  SenseQDDot=off  SenseRDDot=off  SenseX=on  SenseY=on  SenseZ=off  SenseRad=off  SenseAzim=off  SenseDist=off  SenseInc=off  SenseXDot=on  SenseYDot=on  SenseZDot=off  SenseRadDot=off  SenseAzimDot=off  SenseDistDot=off  SenseIncDot=off  SenseXDDot=off  SenseYDDot=off  SenseZDDot=off  SenseRadDDot=off  SenseAzimDDot=off  SenseDistDDot=off  SenseIncDDot=off
  World Frame : sm_lib/Frames and Transforms/World Frame
  contact? : simulink/Logic and Bit Operations/Compare To Zero  relop=<=  OutDataTypeStr=boolean
  Toe : PMIOPort  Side=Right
  GRF : PMIOPort  Port=2  Side=Right
  tag scope: GC_l=global
  wires:
  PS-Simulink Converter/1 -> contact?/1, Ground Friction Model/1(dy [m])  "yBall left"
  contact?/1 -> Ground Friction Model/Enable, [GC_l]
  Ground Friction Model/3(Stiction!) -> Terminator/1
  PS-Simulink Converter3/1 -> Ground Friction Model/4(vx [m/s])
  PS-Simulink Converter2/1 -> Ground Friction Model/3(x [m])
  PS-Simulink Converter1/1 -> Ground Friction Model/2(vy [m/s])
  Ground Friction Model/2(Fx_Friction [N]) -> Simulink-PS Converter/1
  Ground Friction Model/1(Fy_Ground[N]) -> Scope/1, Simulink-PS Converter1/1
  connections:
  Transform Sensor/RConn2 -- PS-Simulink Converter2/LConn1
  External Force and Torque/RConn1 -- GRF/RConn1
  Transform Sensor/RConn1 -- Toe/RConn1
  Transform Sensor/RConn3 -- PS-Simulink Converter/LConn1
  Transform Sensor/RConn5 -- PS-Simulink Converter1/LConn1
  Transform Sensor/LConn1 -- World Frame/RConn1
  Transform Sensor/RConn4 -- PS-Simulink Converter3/LConn1
  External Force and Torque/LConn2 -- Simulink-PS Converter1/RConn1
  External Force and Torque/LConn1 -- Simulink-PS Converter/RConn1

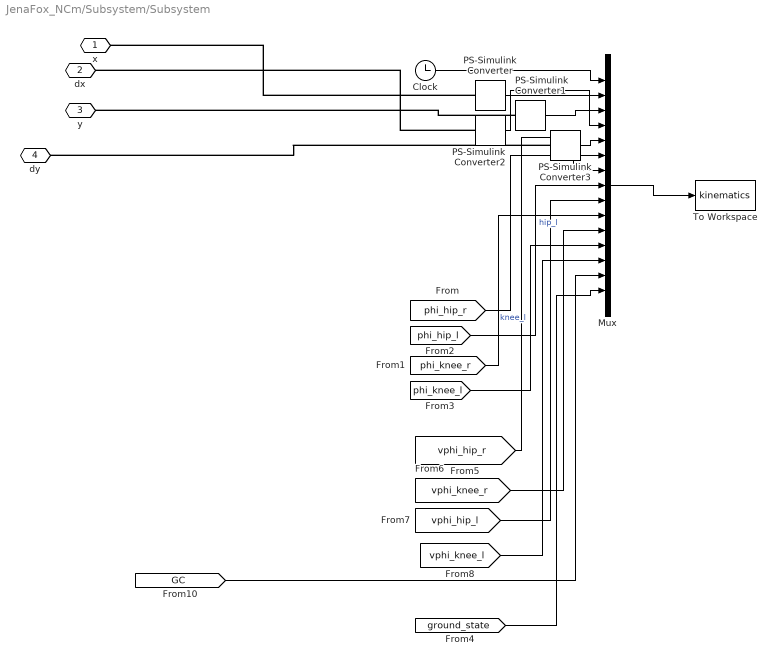
== system JenaFox_NCm/Subsystem/Subsystem ==
  Clock : Clock
  Mux : Mux  Inputs=15
  PS-Simulink Converter{,1..3} (4 alike) : nesl_utility/PS-Simulink Converter  PhysicalDomain=network_engine_domain  SubClassName=ps_output  LeftPortType=input  RightPortType=output  PseudoPeriodic=off  Frequencies=[]  Unit=1  AffineConversion=off
  To Workspace : ToWorkspace  VariableName=kinematics  SampleTime=1e-3
  x : PMIOPort  Side=Left
  dx : PMIOPort  Port=2  Side=Left
  y : PMIOPort  Port=3  Side=Left
  dy : PMIOPort  Port=4  Side=Left
  wires:
  [phi_hip_r] -> Mux/6
  [vphi_knee_l] -> Mux/13
  PS-Simulink Converter3/1 -> Mux/5
  [vphi_hip_l] -> Mux/9
  [phi_hip_l] -> Mux/8  "hip_l"
  [GC] -> Mux/14
  Clock/1 -> Mux/1
  [ground_state] -> Mux/15
  [vphi_hip_r] -> Mux/7
  [phi_knee_r] -> Mux/10
  PS-Simulink Converter1/1 -> Mux/3
  [vphi_knee_r] -> Mux/11
  [phi_knee_l] -> Mux/12  "knee_l"
  PS-Simulink Converter2/1 -> Mux/4
  PS-Simulink Converter/1 -> Mux/2
  Mux/1 -> To Workspace/1
  connections:
  PS-Simulink Converter2/LConn1 -- dx/RConn1
  PS-Simulink Converter1/LConn1 -- y/RConn1
  PS-Simulink Converter/LConn1 -- x/RConn1
  PS-Simulink Converter3/LConn1 -- dy/RConn1

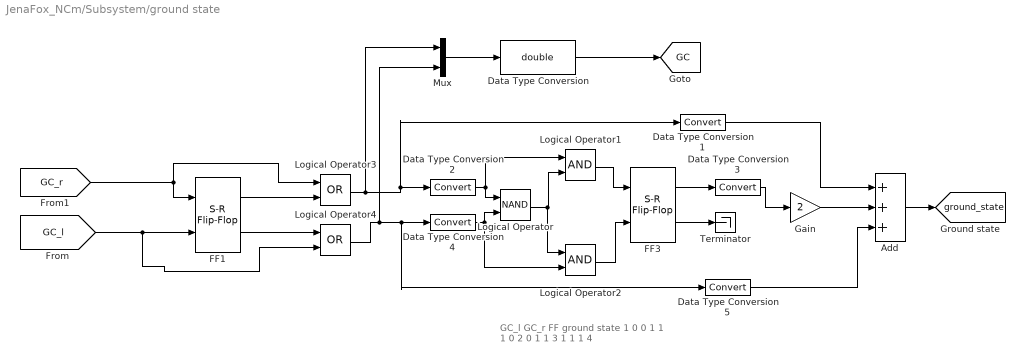
== system JenaFox_NCm/Subsystem/ground state ==
  note: GC_l   GC_r   FF   ground state
      | 1         0         0       1
      | 1         1         0       2
      | 0         1         1       3
      | 1         1         1       4
  Add : Sum  Inputs=+++
  Data Type Conversion : DataTypeConversion  OutDataTypeStr=double
  Data Type Conversion{1..5} (5 alike) : DataTypeConversion
  FF1 : simulink_extras/Flip Flops/S-R Flip-Flop  initial_condition=0
  FF3 : simulink_extras/Flip Flops/S-R Flip-Flop  initial_condition=0
  Gain : Gain  Gain=2
  Logical Operator : Logic  Operator=NAND  AllPortsSameDT=off  OutDataTypeStr=boolean
  Logical Operator1 : Logic  AllPortsSameDT=off  OutDataTypeStr=boolean
  Logical Operator2 : Logic  AllPortsSameDT=off  OutDataTypeStr=boolean
  Logical Operator3 : Logic  Operator=OR  AllPortsSameDT=off  OutDataTypeStr=boolean
  Logical Operator4 : Logic  Operator=OR  AllPortsSameDT=off  OutDataTypeStr=boolean
  Mux : Mux  Inputs=2
  Terminator : Terminator
  tag scope: GC=global, ground_state=global
  wires:
  [GC_l] -> Logical Operator4/2, FF1/2
  [GC_r] -> FF1/1, Logical Operator3/1
  Logical Operator1/1 -> FF3/1
  Data Type Conversion4/1 -> Logical Operator2/2, Logical Operator/2
  Data Type Conversion2/1 -> Logical Operator1/1, Logical Operator/1
  Data Type Conversion3/1 -> Gain/1
  Logical Operator2/1 -> FF3/2
  FF3/2 -> Terminator/1
  FF3/1 -> Data Type Conversion3/1
  Logical Operator/1 -> Logical Operator2/1, Logical Operator1/2
  Gain/1 -> Add/2
  Add/1 -> [ground_state]
  FF1/1 -> Logical Operator3/2
  FF1/2 -> Logical Operator4/1
  Logical Operator4/1 -> Mux/2, Data Type Conversion5/1, Data Type Conversion4/1
  Logical Operator3/1 -> Mux/1, Data Type Conversion1/1, Data Type Conversion2/1
  Mux/1 -> Data Type Conversion/1
  Data Type Conversion/1 -> [GC]
  Data Type Conversion1/1 -> Add/1
  Data Type Conversion5/1 -> Add/3

== system JenaFox_NCm/Subsystem/hip_l ==
  Gain : Gain  Gain=-180/pi
  Gain1 : Gain  Gain=-1
  Gain2 : Gain  Gain=-1
  PS-Simulink Converter1 : nesl_utility/PS-Simulink Converter  PhysicalDomain=network_engine_domain  SubClassName=ps_output  LeftPortType=input  RightPortType=output  PseudoPeriodic=off  Frequencies=[]  Unit=1  AffineConversion=off
  PS-Simulink Converter2 : nesl_utility/PS-Simulink Converter  PhysicalDomain=network_engine_domain  SubClassName=ps_output  LeftPortType=input  RightPortType=output  PseudoPeriodic=off  Frequencies=[]  Unit=1  AffineConversion=off
  Simulink-PS Converter : nesl_utility/Simulink-PS Converter  PhysicalDomain=network_engine_domain  SubClassName=ps_input  LeftPortType=input  RightPortType=output  PseudoPeriodic=off  Frequencies=[]  NoiseDistribution=none  NoiseParameters=[]  Unit=1  AffineConversion=off  FilteringAndDerivatives=provide  SimscapeFilterOrder=1  InputFilterTimeConstant=0.001  UdotUserProvided=0
  hip_l : sm_lib/Joints/Revolute Joint  SenseConstraintForce=off  SenseConstraintForceX=off  SenseConstraintForceY=off  SenseConstraintForceZ=off  SenseConstraintTorque=off  SenseConstraintTorqueX=off  SenseConstraintTorqueY=off  SenseConstraintTorqueZ=off  SenseTotalForce=off  SenseTotalForceX=off  SenseTotalForceY=off  SenseTotalForceZ=off  SenseTotalTorque=off  SenseTotalTorqueX=off  SenseTotalTorqueY=off  SenseTotalTorqueZ=off  CompositeWrenchDir=FollowerOnBase  CompositeWrenchFrame=BaseFrame  EquilibriumPosition=0  EquilibriumPositionUnits=rad  SpringStiffness=0  SpringStiffnessUnits=N*m/rad  DampingCoefficient=d_joint  DampingCoefficientUnits=N*m/(rad/s)  TorqueActuationMode=InputTorque  MotionActuationMode=ComputedMotion  SensePosition=on  SenseVelocity=on  SenseAcceleration=off  SenseTorqueForce=off  PositionTargetSpecify=on  PositionTargetPriority=High  PositionTargetValue=-IC_phi_hip_l  PositionTargetValueUnits=deg  VelocityTargetSpecify=off  VelocityTargetPriority=High  VelocityTargetValue=0  VelocityTargetValueUnits=deg/s
  trunk : PMIOPort  Side=Left
  thigh : PMIOPort  Port=2  Side=Right
  tag scope: phi_hip_l=global, vphi_hip_l=global
  wires:
  PS-Simulink Converter1/1 -> Gain1/1
  [T_hip_l] -> Gain2/1
  PS-Simulink Converter2/1 -> Gain/1
  Gain/1 -> [phi_hip_l]
  Gain1/1 -> [vphi_hip_l]
  Gain2/1 -> Simulink-PS Converter/1
  connections:
  hip_l/RConn2 -- PS-Simulink Converter2/LConn1
  hip_l/RConn1 -- thigh/RConn1
  hip_l/LConn2 -- Simulink-PS Converter/RConn1
  hip_l/RConn3 -- PS-Simulink Converter1/LConn1
  hip_l/LConn1 -- trunk/RConn1

== system JenaFox_NCm/Subsystem/hip_r ==
  Gain : Gain  Gain=-180/pi
  Gain1 : Gain  Gain=-1
  Gain2 : Gain  Gain=-1
  PS-Simulink Converter1 : nesl_utility/PS-Simulink Converter  PhysicalDomain=network_engine_domain  SubClassName=ps_output  LeftPortType=input  RightPortType=output  PseudoPeriodic=off  Frequencies=[]  Unit=1  AffineConversion=off
  PS-Simulink Converter2 : nesl_utility/PS-Simulink Converter  PhysicalDomain=network_engine_domain  SubClassName=ps_output  LeftPortType=input  RightPortType=output  PseudoPeriodic=off  Frequencies=[]  Unit=1  AffineConversion=off
  Simulink-PS Converter : nesl_utility/Simulink-PS Converter  PhysicalDomain=network_engine_domain  SubClassName=ps_input  LeftPortType=input  RightPortType=output  PseudoPeriodic=off  Frequencies=[]  NoiseDistribution=none  NoiseParameters=[]  Unit=1  AffineConversion=off  FilteringAndDerivatives=provide  SimscapeFilterOrder=1  InputFilterTimeConstant=0.001  UdotUserProvided=0
  hip_r : sm_lib/Joints/Revolute Joint  SenseConstraintForce=off  SenseConstraintForceX=off  SenseConstraintForceY=off  SenseConstraintForceZ=off  SenseConstraintTorque=off  SenseConstraintTorqueX=off  SenseConstraintTorqueY=off  SenseConstraintTorqueZ=off  SenseTotalForce=off  SenseTotalForceX=off  SenseTotalForceY=off  SenseTotalForceZ=off  SenseTotalTorque=off  SenseTotalTorqueX=off  SenseTotalTorqueY=off  SenseTotalTorqueZ=off  CompositeWrenchDir=FollowerOnBase  CompositeWrenchFrame=BaseFrame  EquilibriumPosition=0  EquilibriumPositionUnits=rad  SpringStiffness=0  SpringStiffnessUnits=N*m/rad  DampingCoefficient=d_joint  DampingCoefficientUnits=N*m/(rad/s)  TorqueActuationMode=InputTorque  MotionActuationMode=ComputedMotion  SensePosition=on  SenseVelocity=on  SenseAcceleration=off  SenseTorqueForce=off  PositionTargetSpecify=on  PositionTargetPriority=High  PositionTargetValue=-IC_phi_hip_r  PositionTargetValueUnits=deg  VelocityTargetSpecify=off  VelocityTargetPriority=High  VelocityTargetValue=0  VelocityTargetValueUnits=deg/s
  trunk : PMIOPort  Side=Left
  thigh : PMIOPort  Port=2  Side=Right
  tag scope: phi_hip_r=global, vphi_hip_r=global
  wires:
  PS-Simulink Converter1/1 -> Gain1/1
  [T_hip_r] -> Gain2/1
  PS-Simulink Converter2/1 -> Gain/1
  Gain/1 -> [phi_hip_r]
  Gain1/1 -> [vphi_hip_r]
  Gain2/1 -> Simulink-PS Converter/1
  connections:
  hip_r/RConn2 -- PS-Simulink Converter2/LConn1
  hip_r/RConn1 -- thigh/RConn1
  hip_r/LConn2 -- Simulink-PS Converter/RConn1
  hip_r/RConn3 -- PS-Simulink Converter1/LConn1
  hip_r/LConn1 -- trunk/RConn1

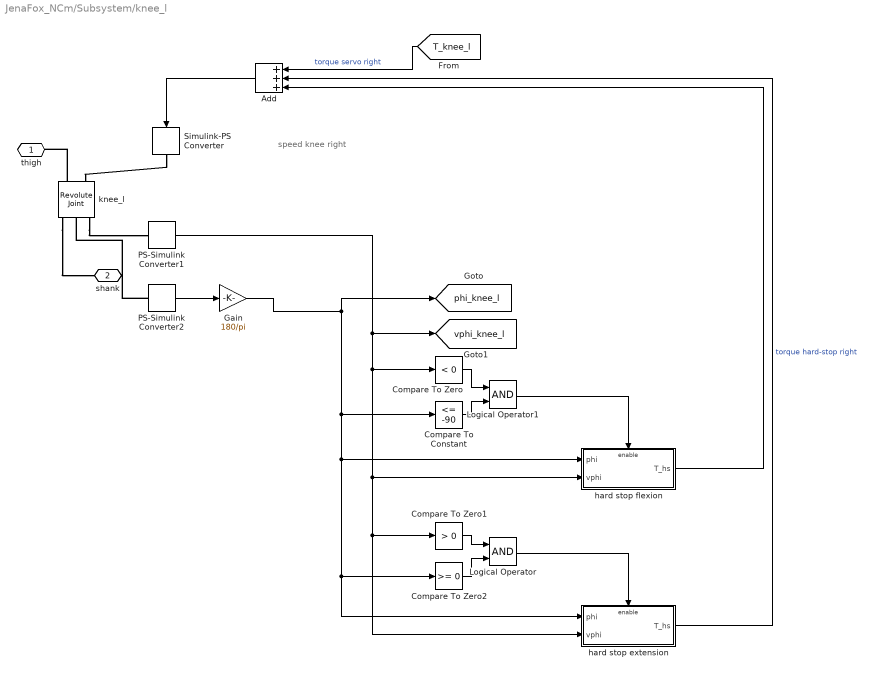
== system JenaFox_NCm/Subsystem/knee_l ==
  note: speed knee right
  Add : Sum  Inputs=+++
  Compare To Constant : simulink/Logic and Bit Operations/Compare To Constant  relop=<=  const=-90  OutDataTypeStr=uint8
  Compare To Zero : simulink/Logic and Bit Operations/Compare To Zero  relop=<  OutDataTypeStr=uint8  ZeroCross=off
  Compare To Zero1 : simulink/Logic and Bit Operations/Compare To Zero  relop=>  OutDataTypeStr=uint8  ZeroCross=off
  Compare To Zero2 : simulink/Logic and Bit Operations/Compare To Zero  relop=>=  OutDataTypeStr=uint8
  Gain : Gain  Gain=180/pi
  Logical Operator : Logic  AllPortsSameDT=off  OutDataTypeStr=boolean
  Logical Operator1 : Logic  AllPortsSameDT=off  OutDataTypeStr=boolean
  PS-Simulink Converter1 : nesl_utility/PS-Simulink Converter  PhysicalDomain=network_engine_domain  SubClassName=ps_output  LeftPortType=input  RightPortType=output  PseudoPeriodic=off  Frequencies=[]  Unit=1  AffineConversion=off
  PS-Simulink Converter2 : nesl_utility/PS-Simulink Converter  PhysicalDomain=network_engine_domain  SubClassName=ps_output  LeftPortType=input  RightPortType=output  PseudoPeriodic=off  Frequencies=[]  Unit=1  AffineConversion=off
  Simulink-PS Converter : nesl_utility/Simulink-PS Converter  PhysicalDomain=network_engine_domain  SubClassName=ps_input  LeftPortType=input  RightPortType=output  PseudoPeriodic=off  Frequencies=[]  NoiseDistribution=none  NoiseParameters=[]  Unit=1  AffineConversion=off  FilteringAndDerivatives=provide  SimscapeFilterOrder=1  InputFilterTimeConstant=0.001  UdotUserProvided=0
  hard stop extension : Subsystem  TreatAsAtomicUnit=on
  hard stop flexion : Subsystem  TreatAsAtomicUnit=on
  knee_l : sm_lib/Joints/Revolute Joint  SenseConstraintForce=off  SenseConstraintForceX=off  SenseConstraintForceY=off  SenseConstraintForceZ=off  SenseConstraintTorque=off  SenseConstraintTorqueX=off  SenseConstraintTorqueY=off  SenseConstraintTorqueZ=off  SenseTotalForce=off  SenseTotalForceX=off  SenseTotalForceY=off  SenseTotalForceZ=off  SenseTotalTorque=off  SenseTotalTorqueX=off  SenseTotalTorqueY=off  SenseTotalTorqueZ=off  CompositeWrenchDir=FollowerOnBase  CompositeWrenchFrame=BaseFrame  EquilibriumPosition=0  EquilibriumPositionUnits=rad  SpringStiffness=0  SpringStiffnessUnits=N*m/rad  DampingCoefficient=d_joint  DampingCoefficientUnits=N*m/(rad/s)  TorqueActuationMode=InputTorque  MotionActuationMode=ComputedMotion  SensePosition=on  SenseVelocity=on  SenseAcceleration=off  SenseTorqueForce=off  PositionTargetSpecify=on  PositionTargetPriority=High  PositionTargetValue=IC_phi_knee_l  PositionTargetValueUnits=deg  VelocityTargetSpecify=off  VelocityTargetPriority=High  VelocityTargetValue=0  VelocityTargetValueUnits=deg/s
  thigh : PMIOPort  Side=Left
  shank : PMIOPort  Port=2  Side=Right
  tag scope: phi_knee_l=global, vphi_knee_l=global
  wires:
  Compare To Constant/1 -> Logical Operator1/2
  PS-Simulink Converter2/1 -> Gain/1
  hard stop extension/1(T_hs) -> Add/2  "torque hard-stop right"
  Compare To Zero1/1 -> Logical Operator/1
  Logical Operator1/1 -> hard stop flexion/Enable
  Logical Operator/1 -> hard stop extension/Enable
  Add/1 -> Simulink-PS Converter/1
  Compare To Zero/1 -> Logical Operator1/1
  PS-Simulink Converter1/1 -> [vphi_knee_l], Compare To Zero/1, hard stop flexion/2(vphi), Compare To Zero1/1, hard stop extension/2(vphi)
  hard stop flexion/1(T_hs) -> Add/3
  Compare To Zero2/1 -> Logical Operator/2
  [T_knee_l] -> Add/1  "torque servo right"
  Gain/1 -> [phi_knee_l], Compare To Constant/1, hard stop flexion/1(phi), Compare To Zero2/1, hard stop extension/1(phi)
  connections:
  Simulink-PS Converter/RConn1 -- knee_l/LConn2
  knee_l/RConn1 -- shank/RConn1
  PS-Simulink Converter2/LConn1 -- knee_l/RConn2
  knee_l/RConn3 -- PS-Simulink Converter1/LConn1
  knee_l/LConn1 -- thigh/RConn1
